simulink model "sampleModel1778"  (R2023a)
settings: Solver=VariableStepAuto  StartTime=0.0  StopTime=10.0  RelTol=1e-3
libraries: simulink x3, hdlsllib x3
settings Model: Creator=user1  LastModifiedBy=user1

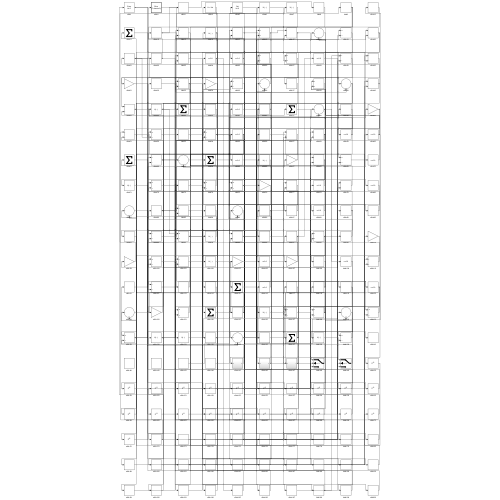
[thumbnail: Simulink's stored preview of the top-level diagram]
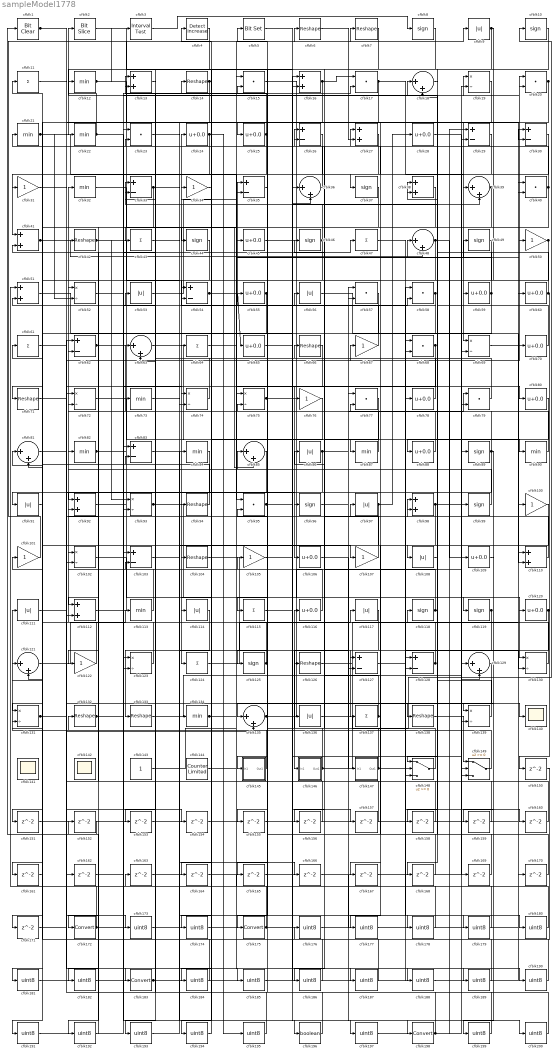
== system sampleModel1778 ==
  cfblk1 : simulink/Logic and Bit Operations/Bit Clear  iBit=0
      settings: LibrarySourceBlock=|
      | hdlsllib/Logic and Bit
      | Operations/Bit Clear
  cfblk{8,10,37,44,46,49,89,96,99,118..119,125} (12 alike) : Signum
  cfblk{31,34,50,67,76,100..101,105,107,122} (10 alike) : Gain
  cfblk{19,52,69,72,74..75,93,102,123,130..131,139} (12 alike) : Product  Inputs=*/  RndMeth=Zero  SaturateOnIntegerOverflow=on
  cfblk{26,29..30,33,35,54,62,83,103,127..128} (11 alike) : Sum  Inputs=+-
  cfblk{6..7,14,42,66,71,94,104,126,132..133,138} (12 alike) : Reshape
  cfblk{24..25,28,45,55,59..60,65,70,78,80,88,106,109,116,120} (16 alike) : Bias  Bias=0.0  SaturateOnIntegerOverflow=off
  cfblk{9,53,56,86,91,97,108,111,114,117,136} (11 alike) : Abs  SaturateOnIntegerOverflow=off
  cfblk{11,43,47,61,64,115,124,137} (8 alike) : Sum  Inputs=+
  cfblk{13,16,27,38,41,51,92,98,110,112} (10 alike) : Sum
  cfblk{12,21..22,32,73,82,84,87,90,113,134} (11 alike) : MinMax
  cfblk{18,36,39,48,63,81,85,121,129,135} (10 alike) : Sum  Inputs=|++
  cfblk140 : Scope
  cfblk141 : Scope
      settings: Floating=on
  cfblk142 : Scope
      settings: Floating=on
  cfblk143 : Constant  SampleTime=-1
  cfblk144 : hdlsllib/Sources/Counter Limited  uplimit=7  tsamp=-1
  cfblk145 : Subsystem
      settings: LibrarySourceBlock=|
      | hdlsllib/Ports &
      | Subsystems/Subsystem
  cfblk146 : Subsystem
      settings: LibrarySourceBlock=|
      | hdlsllib/Ports &
      | Subsystems/Subsystem
  cfblk147 : Subsystem
      settings: LibrarySourceBlock=|
      | hdlsllib/Ports &
      | Subsystems/Subsystem
  cfblk148 : Switch  SaturateOnIntegerOverflow=off  InputSameDT=off
  cfblk149 : Switch  SaturateOnIntegerOverflow=off  InputSameDT=off
  cfblk{15,17,20,23,40,57..58,68,77,79,95} (11 alike) : DotProduct  OutDataTypeStr=Inherit: Inherit via internal rule
  cfblk{150..171} (22 alike) : Delay  SampleTime=1
  cfblk{172,175,183,198} (4 alike) : DataTypeConversion  SaturateOnIntegerOverflow=off  RndMeth=Floor
  cfblk{173..174,176..182,184..195,197,199..200} (24 alike) : DataTypeConversion  OutDataTypeStr=uint8  SaturateOnIntegerOverflow=off  RndMeth=Floor
  cfblk196 : DataTypeConversion  OutDataTypeStr=boolean  SaturateOnIntegerOverflow=off  RndMeth=Floor
  cfblk2 : hdlsllib/Logic and Bit Operations/Bit Slice  lidx=7  ridx=0
  cfblk3 : hdlsllib/Logic and Bit Operations/Interval Test  IntervalClosedRight=on  uplimit=0.5  IntervalClosedLeft=on  lowlimit=-0.5  OutDataTypeStr=boolean
  cfblk4 : simulink/Logic and Bit Operations/Detect Increase  vinit=0.0  OutDataTypeStr=boolean
      settings: LibrarySourceBlock=|
      | hdlsllib/Logic and Bit
      | Operations/Detect
      | Increase
  cfblk5 : simulink/Logic and Bit Operations/Bit Set  iBit=0
      settings: LibrarySourceBlock=|
      | hdlsllib/Logic and Bit
      | Operations/Bit Set
  wires:
  cfblk145/1(Out1) -> cfblk111/1
  cfblk48/1 -> cfblk109/1, cfblk148/3
  cfblk124/1 -> cfblk117/1
  cfblk45/1 -> cfblk130/1
  cfblk24/1 -> cfblk41/1, cfblk195/1
  cfblk122/1 -> cfblk32/1
  cfblk68/1 -> cfblk106/1, cfblk93/2
  cfblk114/1 -> cfblk133/1
  cfblk129/1 -> cfblk175/1
  cfblk37/1 -> cfblk85/2
  cfblk78/1 -> cfblk41/2
  cfblk101/1 -> cfblk6/1
  cfblk49/1 -> cfblk124/1
  cfblk69/1 -> cfblk20/1
  cfblk112/1 -> cfblk7/1
  cfblk133/1 -> cfblk89/1
  cfblk9/1 -> cfblk125/1, cfblk18/2, cfblk59/1
  cfblk35/1 -> cfblk145/1(In1)
  cfblk135/1 -> cfblk99/1, cfblk39/2
  cfblk54/1 -> cfblk65/1, cfblk80/1
  cfblk25/1 -> cfblk13/1, cfblk71/1
  cfblk67/1 -> cfblk35/1
  cfblk149/1 -> cfblk132/1
  cfblk74/1 -> cfblk53/1
  cfblk12/1 -> cfblk69/1, cfblk3/1
  cfblk113/1 -> cfblk52/1
  cfblk57/1 -> cfblk172/1
  cfblk99/1 -> cfblk82/1
  cfblk46/1 -> cfblk121/2, cfblk13/2
  cfblk52/1 -> cfblk20/2
  cfblk126/1 -> cfblk60/1
  cfblk83/1 -> cfblk198/1
  cfblk97/1 -> cfblk135/1, cfblk28/1
  cfblk138/1 -> cfblk149/1
  cfblk38/1 -> cfblk92/1
  cfblk93/1 -> cfblk119/1, cfblk127/2
  cfblk137/1 -> cfblk27/1, cfblk26/2
  cfblk16/1 -> cfblk17/1, cfblk25/1
  cfblk55/1 -> cfblk153/1, cfblk193/1
  cfblk50/1 -> cfblk94/1, cfblk139/2
  cfblk62/1 -> cfblk24/1, cfblk196/1
  cfblk136/1 -> cfblk10/1
  cfblk92/1 -> cfblk58/2
  cfblk98/1 -> cfblk69/2, cfblk167/1
  cfblk132/1 -> cfblk47/1, cfblk54/1
  cfblk15/1 -> cfblk87/1
  cfblk60/1 -> cfblk38/1, cfblk33/2, cfblk150/1
  cfblk53/1 -> cfblk35/2
  cfblk6/1 -> cfblk27/2
  cfblk131/1 -> cfblk67/1, cfblk140/1
  cfblk75/1 -> cfblk149/3, cfblk165/1
  cfblk22/1 -> cfblk2/1, cfblk189/1
  cfblk81/1 -> cfblk96/1
  cfblk21/1 -> cfblk95/1, cfblk52/2, cfblk135/2
  cfblk20/1 -> cfblk88/1, cfblk31/1
  cfblk82/1 -> cfblk70/1, cfblk42/1, cfblk17/2
  cfblk107/1 -> cfblk66/1
  cfblk63/1 -> cfblk128/1
  cfblk118/1 -> cfblk56/1, cfblk38/2
  cfblk4/1 -> cfblk22/1
  cfblk146/1(Out1) -> cfblk78/1, cfblk72/2
  cfblk116/1 -> cfblk102/1
  cfblk110/1 -> cfblk98/1
  cfblk8/1 -> cfblk44/1
  cfblk106/1 -> cfblk147/1(In1)
  cfblk147/1(Out1) -> cfblk116/1, cfblk180/1
  cfblk43/1 -> cfblk107/1
  cfblk47/1 -> cfblk130/2
  cfblk2/1 -> cfblk36/2
  cfblk120/1 -> cfblk139/1, cfblk177/1
  cfblk128/1 -> cfblk46/1, cfblk127/1
  cfblk121/1 -> cfblk113/1
  cfblk143/1 -> cfblk98/2
  cfblk115/1 -> cfblk19/1
  cfblk58/1 -> cfblk131/1, cfblk54/2
  cfblk134/1 -> cfblk9/1, cfblk164/1
  cfblk44/1 -> cfblk112/1
  cfblk70/1 -> cfblk18/1
  cfblk119/1 -> cfblk137/1, cfblk168/1
  cfblk56/1 -> cfblk110/2
  cfblk90/1 -> cfblk63/1
  cfblk41/1 -> cfblk48/2, cfblk81/2
  cfblk42/1 -> cfblk134/1, cfblk93/1
  cfblk94/1 -> cfblk11/1
  cfblk66/1 -> cfblk114/1
  cfblk87/1 -> cfblk62/2
  cfblk104/1 -> cfblk146/1(In1)
  cfblk14/1 -> cfblk104/1, cfblk74/2
  cfblk10/1 -> cfblk63/2
  cfblk95/1 -> cfblk49/1, cfblk179/1
  cfblk40/1 -> cfblk4/1, cfblk171/1
  cfblk123/1 -> cfblk81/1
  cfblk39/1 -> cfblk138/1, cfblk161/1
  cfblk17/1 -> cfblk64/1, cfblk39/1
  cfblk148/1 -> cfblk86/1
  cfblk117/1 -> cfblk126/1
  cfblk59/1 -> cfblk12/1, cfblk45/1, cfblk191/1
  cfblk86/1 -> cfblk91/1, cfblk79/1
  cfblk108/1 -> cfblk148/1
  cfblk36/1 -> cfblk21/1
  cfblk18/1 -> cfblk108/1
  cfblk89/1 -> cfblk26/1, cfblk159/1, cfblk174/1
  cfblk79/1 -> cfblk51/2
  cfblk130/1 -> cfblk101/1
  cfblk51/1 -> cfblk76/1
  cfblk139/1 -> cfblk118/1
  cfblk29/1 -> cfblk123/2
  cfblk19/1 -> cfblk37/1
  cfblk111/1 -> cfblk97/1
  cfblk64/1 -> cfblk90/1
  cfblk13/1 -> cfblk43/1
  cfblk3/1 -> cfblk8/1
  cfblk102/1 -> cfblk120/1
  cfblk32/1 -> cfblk75/1
  cfblk125/1 -> cfblk33/1, cfblk75/2
  cfblk144/1 -> cfblk50/1
  cfblk88/1 -> cfblk55/1
  cfblk61/1 -> cfblk183/1
  cfblk30/1 -> cfblk115/1
  cfblk72/1 -> cfblk136/1
  cfblk96/1 -> cfblk77/1
  cfblk27/1 -> cfblk112/2
  cfblk1/1 -> cfblk30/2, cfblk74/1
  cfblk33/1 -> cfblk122/1, cfblk166/1
  cfblk91/1 -> cfblk151/1
  cfblk151/1 -> cfblk30/1
  cfblk152/1 -> cfblk1/1
  cfblk153/1 -> cfblk148/2
  cfblk31/1 -> cfblk154/1
  cfblk154/1 -> cfblk58/1
  cfblk26/1 -> cfblk155/1
  cfblk155/1 -> cfblk128/2
  cfblk7/1 -> cfblk156/1
  cfblk156/1 -> cfblk62/1
  cfblk65/1 -> cfblk157/1
  cfblk157/1 -> cfblk85/1
  cfblk80/1 -> cfblk158/1
  cfblk158/1 -> cfblk16/1
  cfblk159/1 -> cfblk95/2
  cfblk127/1 -> cfblk160/1
  cfblk160/1 -> cfblk92/2
  cfblk161/1 -> cfblk131/2
  cfblk71/1 -> cfblk162/1
  cfblk162/1 -> cfblk123/1
  cfblk163/1 -> cfblk68/2
  cfblk165/1 -> cfblk36/1
  cfblk167/1 -> cfblk19/2
  cfblk168/1 -> cfblk77/2
  cfblk28/1 -> cfblk169/1
  cfblk169/1 -> cfblk48/1
  cfblk170/1 -> cfblk15/2
  cfblk171/1 -> cfblk102/2
  cfblk172/1 -> cfblk149/2, cfblk121/1
  cfblk11/1 -> cfblk173/1
  cfblk173/1 -> cfblk57/1
  cfblk174/1 -> cfblk57/2
  cfblk175/1 -> cfblk79/2, cfblk40/2, cfblk15/1
  cfblk150/1 -> cfblk176/1
  cfblk176/1 -> cfblk129/1
  cfblk177/1 -> cfblk129/2
  cfblk103/1 -> cfblk178/1
  cfblk178/1 -> cfblk51/1
  cfblk179/1 -> cfblk103/1
  cfblk180/1 -> cfblk103/2
  cfblk100/1 -> cfblk181/1
  cfblk181/1 -> cfblk68/1
  cfblk85/1 -> cfblk182/1
  cfblk182/1 -> cfblk100/1
  cfblk183/1 -> cfblk163/1, cfblk16/2
  cfblk76/1 -> cfblk184/1
  cfblk184/1 -> cfblk61/1
  cfblk23/1 -> cfblk185/1
  cfblk185/1 -> cfblk40/1
  cfblk77/1 -> cfblk186/1
  cfblk186/1 -> cfblk23/1
  cfblk164/1 -> cfblk187/1
  cfblk187/1 -> cfblk23/2
  cfblk105/1 -> cfblk188/1
  cfblk188/1 -> cfblk170/1
  cfblk189/1 -> cfblk105/1
  cfblk73/1 -> cfblk190/1
  cfblk190/1 -> cfblk110/1
  cfblk191/1 -> cfblk73/1
  cfblk84/1 -> cfblk192/1
  cfblk192/1 -> cfblk152/1
  cfblk193/1 -> cfblk84/1
  cfblk34/1 -> cfblk194/1
  cfblk194/1 -> cfblk14/1
  cfblk195/1 -> cfblk34/1
  cfblk196/1 -> cfblk5/1
  cfblk5/1 -> cfblk197/1
  cfblk197/1 -> cfblk29/2
  cfblk198/1 -> cfblk72/1, cfblk29/1
  cfblk109/1 -> cfblk199/1
  cfblk199/1 -> cfblk83/1
  cfblk166/1 -> cfblk200/1
  cfblk200/1 -> cfblk83/2

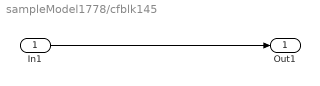
== system sampleModel1778/cfblk145 ==
  In1 : Inport
  Out1 : Outport
  wires:
  In1/1 -> Out1/1

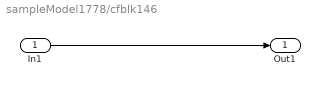
== system sampleModel1778/cfblk146 ==
  In1 : Inport
  Out1 : Outport
  wires:
  In1/1 -> Out1/1

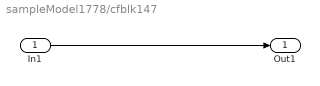
== system sampleModel1778/cfblk147 ==
  In1 : Inport
  Out1 : Outport
  wires:
  In1/1 -> Out1/1
